simulink model "AFMss_fp_obshas_uk_threeaxis"  (R2018a)
settings: Solver=ode4  StartTime=0.0  StopTime=trun  FixedStep=Ts  RelTol=1e-5  EnableMultiTasking=on
PreLoadFcn:
  | VSS_CONTROL_MODE=1;
  | VSS_LINEAR_CONTROL=Simulink.Variant('VSS_CONTROL_MODE==1');
  | VSS_MPC_CONTROL=Simulink.Variant('VSS_CONTROL_MODE == 2');
  | 
  | 
  | VSS_STATE_DIRECT=Simulink.Variant('VSS_STATE_MODE==1');
  | VSS_STATE_OBS=Simulink.Variant('VSS_STATE_MODE==2');
  | VSS_STATE_DIST_OBS=Simulink.Variant('VSS_STATE_MODE==3');
  | VSS_STATE_MODE=1;
undefined symbols (not defined in the file): C_ydist, Ident_obs, K_lqr, PLANT, sim_obj, Ts, uss_0, x0
libraries: cstblocks x2
settings Model: Creator=arnold  LastModifiedBy=arnold
settings DataIOCC: SaveFormat=Array  SaveOutput=off  SaveState=on  InspectSignalLogs=on  TimeSaveName=tout_ptos
settings OptimizationCC: LifeSpan=inf
settings DebuggingCC: SolverPrmCheckMsg=warning  SFUnexpectedBacktrackingDiag=warning  SFNoUnconditionalDefaultTransitionDiag=warning  SFExecutionAtInitializationDiag=none
settings HardwareCC: ProdBitPerPointer=32  ProdBitPerSizeT=32  ProdBitPerPtrDiffT=32  ProdLargestAtomicFloat=None  ProdIntDivRoundTo=Undefined  ProdEndianess=Unspecified  ProdWordSize=32  ProdHWDeviceType=32-bit Generic
settings ModelReferenceCC: PropagateSignalLabelsOutOfModel=off
settings CodeAppCC: StateflowObjectComments=on
settings GRTTargetCC: TargetLangStandard=C89/C90 (ANSI)  GeneratePreprocessorConditionals=Disable all
settings ConfigComp: CovMetricSettings=dw  CovHtmlReporting=on  CovSaveCumulativeToWorkspaceVar=on  CovSaveSingleToWorkspaceVar=on  CovExternalEMLEnable=off  CovSFcnEnable=off

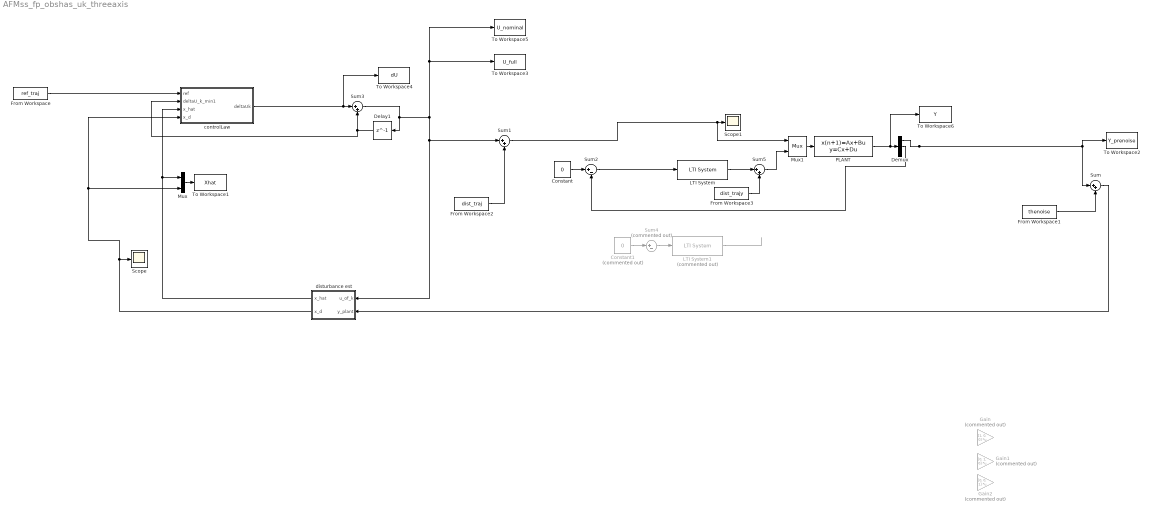
== system AFMss_fp_obshas_uk_threeaxis ==
  Constant : Constant  Value=0
  Constant1 : Constant  Commented=on  Value=0
  Delay1 : Delay  DelayLength=1  InitialCondition=uss_0  SampleTime=Ts
  Demux : Demux  Outputs=3
  From Workspace : FromWorkspace  VariableName=ref_traj  SampleTime=Ts
  From Workspace1 : FromWorkspace  VariableName=thenoise  SampleTime=Ts
  From Workspace2 : FromWorkspace  VariableName=dist_traj  SampleTime=Ts
  From Workspace3 : FromWorkspace  VariableName=dist_trajy  SampleTime=Ts
  Gain : Gain  Commented=on  Gain=[1, 0, 0]  Multiplication=Matrix(K*u)
  Gain1 : Gain  Commented=on  Gain=[0, 1, 0]  Multiplication=Matrix(K*u)
  Gain2 : Gain  Commented=on  Gain=[0, 0, 1]  Multiplication=Matrix(K*u)
  LTI System : cstblocks/LTI System  sys=zpk([0], [1], [0.01], Ts)  IC=[]
  LTI System1 : cstblocks/LTI System  Commented=on  sys=zpk([0], [1], [-0.02], Ts)  IC=[]
  Mux : Mux  Inputs=2
  Mux1 : Mux  Inputs=2
      settings: DisplayOption=signals
  PLANT : DiscreteStateSpace  A=PLANT.a  B=PLANT.b  C=PLANT.c  D=zeros(size(PLANT.c,1), size(PLANT.b, 2))  InitialCondition=x0  SampleTime=Ts
  Scope : Scope
  Scope1 : Scope
  Sum{,1,3,5} (4 alike) : Sum  Inputs=|++
  Sum2 : Sum  Inputs=|+-
  Sum4 : Sum  Commented=on  Inputs=|+-
  To Workspace1 : ToWorkspace  VariableName=Xhat  SaveFormat=Timeseries  SampleTime=-1
      settings: Save2DSignal=2-D array (concatenate along first dimension)
  To Workspace2 : ToWorkspace  VariableName=Y_prenoise  SaveFormat=Timeseries  SampleTime=-1
      settings: Save2DSignal=2-D array (concatenate along first dimension)
  To Workspace3 : ToWorkspace  VariableName=U_full  SaveFormat=Timeseries  SampleTime=-1
      settings: Save2DSignal=2-D array (concatenate along first dimension)
  To Workspace4 : ToWorkspace  VariableName=dU  SaveFormat=Timeseries  SampleTime=-1
      settings: Save2DSignal=2-D array (concatenate along first dimension)
  To Workspace5 : ToWorkspace  VariableName=U_nominal  SaveFormat=Timeseries  SampleTime=-1
      settings: Save2DSignal=2-D array (concatenate along first dimension)
  To Workspace6 : ToWorkspace  VariableName=Y  SaveFormat=Timeseries  SampleTime=-1
      settings: Save2DSignal=2-D array (concatenate along first dimension)
  controlLaw : Subsystem
  disturbance est : Subsystem  VariantControl=VSS_STATE_DIST_OBS
  wires:
  Demux/1 -> To Workspace2/1, Sum/1
  disturbance est/1(x_hat) -> Mux/1, controlLaw/3(x_hat)
  From Workspace1/1 -> Sum/2
  Delay1/1 -> Sum3/2, controlLaw/2(deltaU_k_min1)
  Sum3/1 -> To Workspace3/1, To Workspace5/1, Sum1/1, disturbance est/1(u_of_k), Delay1/1
  controlLaw/1(deltaUk) -> To Workspace4/1, Sum3/1
  From Workspace/1 -> controlLaw/1(ref)
  disturbance est/2(x_d) -> Mux/2, controlLaw/4(x_d), Scope/1
  Mux/1 -> To Workspace1/1
  From Workspace2/1 -> Sum1/2
  Sum/1 -> disturbance est/2(y_plant)
  Sum2/1 -> LTI System/1
  LTI System/1 -> Sum5/1
  Constant/1 -> Sum2/1
  Demux/2 -> Sum2/2
  Sum4/1 -> LTI System1/1
  Constant1/1 -> Sum4/1
  ? -> Sum4/2
  LTI System1/1 -> ?
  ? -> Gain2/1
  ? -> Gain1/1
  ? -> Gain/1
  Sum1/1 -> Mux1/1, Scope1/1
  Mux1/1 -> PLANT/1
  PLANT/1 -> To Workspace6/1, Demux/1
  Sum5/1 -> Mux1/2
  From Workspace3/1 -> Sum5/2

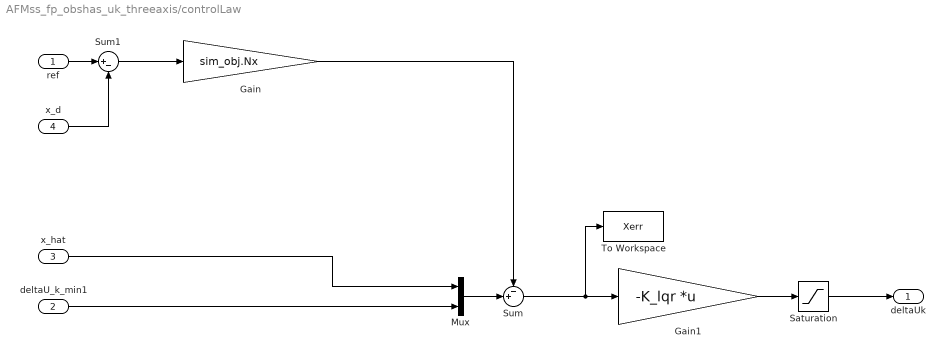
== system AFMss_fp_obshas_uk_threeaxis/controlLaw ==
  ref : Inport
  deltaU_k_min1 : Inport  Port=2
  x_hat : Inport  Port=3
  x_d : Inport  Port=4
  Gain : Gain  Gain=sim_obj.Nx
  Gain1 : Gain  Gain=-K_lqr  Multiplication=Matrix(K*u)
  Mux : Mux  Inputs=2
  Saturation : Saturate  UpperLimit=sim_obj.du_max  LowerLimit=-sim_obj.du_max
  Sum : Sum  Inputs=-+|
  Sum1 : Sum  Inputs=|+-
  To Workspace : ToWorkspace  VariableName=Xerr  SaveFormat=Timeseries  SampleTime=-1
  deltaUk : Outport
  wires:
  Saturation/1 -> deltaUk/1
  Gain1/1 -> Saturation/1
  ref/1 -> Sum1/1
  Sum/1 -> Gain1/1, To Workspace/1
  x_hat/1 -> Mux/1
  deltaU_k_min1/1 -> Mux/2
  Mux/1 -> Sum/2
  Gain/1 -> Sum/1
  Sum1/1 -> Gain/1
  x_d/1 -> Sum1/2

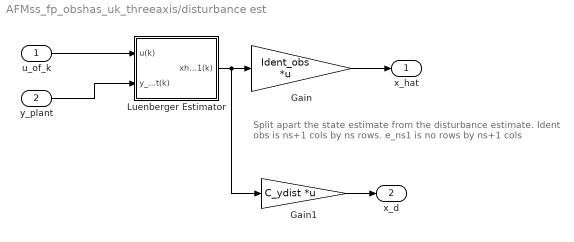
== system AFMss_fp_obshas_uk_threeaxis/disturbance est ==
  note: Split apart the state estimate from the disturbance estimate.
      | Ident obs is ns+1 cols by ns rows. e_ns1 is no rows by ns+1 cols
  u_of_k : Inport
  y_plant : Inport  Port=2
  Gain : Gain  Gain=Ident_obs  Multiplication=Matrix(K*u)
  Gain1 : Gain  Gain=C_ydist  Multiplication=Matrix(K*u)
  Luenberger Estimator : Subsystem  AncestorBlock=customLibFcns/Input Delay Luenberger Estimator
  x_hat : Outport
  x_d : Outport  Port=2
  wires:
  u_of_k/1 -> Luenberger Estimator/1(u(k))
  Luenberger Estimator/1(xhat_1(k)) -> Gain1/1, Gain/1
  y_plant/1 -> Luenberger Estimator/2(y_plant(k))
  Gain/1 -> x_hat/1
  Gain1/1 -> x_d/1

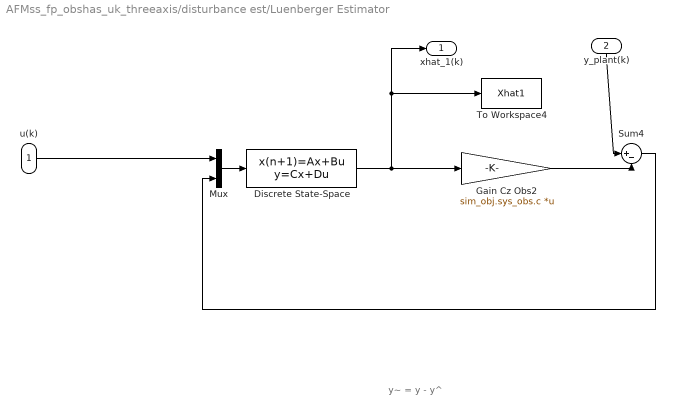
== system AFMss_fp_obshas_uk_threeaxis/disturbance est/Luenberger Estimator ==
  note: y~ = y - y^
  u(k) : Inport
  y_plant(k) : Inport  Port=2
  Discrete State-Space : DiscreteStateSpace  A=sim_obj.sys_obs.a  B=[sim_obj.sys_obs.b, sim_obj.L]  C=eye(length(sim_obj.sys_obs.b))  D=zeros(length(sim_obj.sys_obs.b), 2)  InitialCondition=sim_obj.x0_obs  SampleTime=Ts
  Gain Cz Obs2 : Gain  Gain=sim_obj.sys_obs.c  Multiplication=Matrix(K*u)
  Mux : Mux  Inputs=2
  Sum4 : Sum  Inputs=|+-
  To Workspace4 : ToWorkspace  VariableName=Xhat1  SaveFormat=Timeseries  SampleTime=-1
      settings: Save2DSignal=2-D array (concatenate along first dimension)
  xhat_1(k) : Outport
  wires:
  Sum4/1 -> Mux/2
  u(k)/1 -> Mux/1
  Mux/1 -> Discrete State-Space/1
  Discrete State-Space/1 -> Gain Cz Obs2/1, To Workspace4/1, xhat_1(k)/1
  Gain Cz Obs2/1 -> Sum4/2
  y_plant(k)/1 -> Sum4/1
